simulink model "SPGF_FSK_0000_R2019b"  (R2019b)
settings: Solver=ode3  SolverName=ode4  StartTime=0.0  StopTime=1.4  FixedStep=50e-6/50  RelTol=1e-3  EnableMultiTasking=on
undefined symbols (not defined in the file): D11, Delta
libraries: powerlib x2544, powerlib_meascontrol x204, simulink x24
(part 10 of 33)

== system SPGF_FSK_0000_R2019b/TP42/Nonlinear Load ==
  Cap : powerlib/Elements/Series RLC Branch  LConnTagsString=__new0  RConnTagsString=__new0  BranchType=C  Resistance=34  Inductance=1.04  SetiL0=off  InitialCurrent=0  Capacitance=4e-06  Setx0=off  InitialVoltage=0  Measurements=None
  Cap1 : powerlib/Elements/Series RLC Branch  LConnTagsString=__new0  RConnTagsString=__new0  BranchType=C  Resistance=34  Inductance=1.04  SetiL0=off  InitialCurrent=0  Capacitance=4e-06  Setx0=off  InitialVoltage=0  Measurements=None
  Cap2 : powerlib/Elements/Series RLC Branch  LConnTagsString=__new0  RConnTagsString=__new0  BranchType=C  Resistance=34  Inductance=1.04  SetiL0=off  InitialCurrent=0  Capacitance=4e-06  Setx0=off  InitialVoltage=0  Measurements=None
  Ground : powerlib/Elements/Ground  LConnTagsString=a
  RL : powerlib/Elements/Series RLC Branch  LConnTagsString=__new0  RConnTagsString=__new0  BranchType=RL  Resistance=58  Inductance=1.04  SetiL0=off  InitialCurrent=0  Capacitance=1e-6  Setx0=off  InitialVoltage=0  Measurements=None
  RL1 : powerlib/Elements/Series RLC Branch  LConnTagsString=__new0  RConnTagsString=__new0  BranchType=RL  Resistance=40  Inductance=1.04  SetiL0=off  InitialCurrent=0  Capacitance=1e-6  Setx0=off  InitialVoltage=0  Measurements=None
  RL2 : powerlib/Elements/Series RLC Branch  LConnTagsString=__new0  RConnTagsString=__new0  BranchType=RL  Resistance=40  Inductance=1.04  SetiL0=off  InitialCurrent=0  Capacitance=1e-6  Setx0=off  InitialVoltage=0  Measurements=None
  Universal Bridge : powerlib/Power Electronics/Universal Bridge  Arms=2  SnubberResistance=1e5  SnubberCapacitance=inf  Device=Diodes  Ron=1e-3  Lon=0  ForwardVoltages="[  0  0  ]"  ForwardVoltage=-160  GTOparameters=[ 10e-6 , 20e-6 ]  IGBTparameters=[ 1e-6 , 2e-6 ]  Measurements=None  Measurements_2=None  converterType=Rectifier
  Universal Bridge1 : powerlib/Power Electronics/Universal Bridge  Arms=2  SnubberResistance=1e5  SnubberCapacitance=inf  Device=Diodes  Ron=1e-3  Lon=0  ForwardVoltages="[  0  0  ]"  ForwardVoltage=-160  GTOparameters=[ 10e-6 , 20e-6 ]  IGBTparameters=[ 1e-6 , 2e-6 ]  Measurements=None  Measurements_2=None  converterType=Rectifier
  Universal Bridge2 : powerlib/Power Electronics/Universal Bridge  Arms=2  SnubberResistance=1e5  SnubberCapacitance=inf  Device=Diodes  Ron=1e-3  Lon=0  ForwardVoltages="[  0  0  ]"  ForwardVoltage=-160  GTOparameters=[ 10e-6 , 20e-6 ]  IGBTparameters=[ 1e-6 , 2e-6 ]  Measurements=None  Measurements_2=None  converterType=Rectifier
  A : PMIOPort  Side=Left
  B : PMIOPort  Port=2  Side=Left
  C : PMIOPort  Port=3  Side=Left
  connections:
  Cap/LConn1 -- Universal Bridge/RConn1 -- RL/LConn1
  Cap/RConn1 -- RL/RConn1 -- Universal Bridge/RConn2
  Cap1/LConn1 -- Universal Bridge1/RConn1 -- RL1/LConn1
  Universal Bridge1/RConn2 -- RL1/RConn1 -- Cap1/RConn1
  Cap2/LConn1 -- Universal Bridge2/RConn1 -- RL2/LConn1
  Cap2/RConn1 -- Universal Bridge2/RConn2 -- RL2/RConn1
  Universal Bridge/LConn1 -- A/RConn1
  Universal Bridge1/LConn1 -- B/RConn1
  Universal Bridge2/LConn1 -- C/RConn1
  Ground/LConn1 -- Universal Bridge/LConn2 -- Universal Bridge1/LConn2 -- Universal Bridge2/LConn2

== system SPGF_FSK_0000_R2019b/TP42/Nonlinear Load 3ph ==
  Cap : powerlib/Elements/Series RLC Branch  LConnTagsString=__new0  RConnTagsString=__new0  BranchType=C  Resistance=34  Inductance=1.04  SetiL0=off  InitialCurrent=0  Capacitance=4e-06  Setx0=off  InitialVoltage=0  Measurements=None
  RL : powerlib/Elements/Series RLC Branch  LConnTagsString=__new0  RConnTagsString=__new0  BranchType=RL  Resistance=58  Inductance=1.04  SetiL0=off  InitialCurrent=0  Capacitance=1e-6  Setx0=off  InitialVoltage=0  Measurements=None
  Universal Bridge : powerlib/Power Electronics/Universal Bridge  Arms=3  SnubberResistance=1e5  SnubberCapacitance=inf  Device=Diodes  Ron=1e-3  Lon=0  ForwardVoltages="[  0  0  ]"  ForwardVoltage=-160  GTOparameters=[ 10e-6 , 20e-6 ]  IGBTparameters=[ 1e-6 , 2e-6 ]  Measurements=None  Measurements_2=None  converterType=Rectifier
  A : PMIOPort  Side=Left
  B : PMIOPort  Port=2  Side=Left
  C : PMIOPort  Port=3  Side=Left
  connections:
  Universal Bridge/RConn1 -- RL/LConn1 -- Cap/LConn1
  Cap/RConn1 -- Universal Bridge/RConn2 -- RL/RConn1
  Universal Bridge/LConn2 -- B/RConn1
  C/RConn1 -- Universal Bridge/LConn3
  A/RConn1 -- Universal Bridge/LConn1

== system SPGF_FSK_0000_R2019b/TP42/Q ==
  breaker : Subsystem  Commented=on  mask{SwitchA=off, SwitchB=off, SwitchC=off, InitialStatus=[1 1 1], BreakerResistance=0.0001, SnubberResistance=1e6, SnubberCapacitance=inf, TransitionTimes=[0.5 0.7], ShiftTimes=[0 0 0]}
      mask prompts: SwitchA "Switching of phase A"; SwitchB "Switching of phase B"; SwitchC "Switching of phase C"; InitialStatus "Initial status of phase breaker [A, B, C]"; BreakerResistance "Breaker resistance Ron (ohms) :"; SnubberResistance "Snubbers resistance Rp (ohms) :"; SnubberCapacitance "Snubbers capacitance Cp (F) :"; TransitionTimes "Transition times (s) :"; ShiftTimes "Time differences for switch [tA, tB, tC] (s) :"
      mask init: same as SPGF_FSK_0000_R2019b/Feed/Q/breaker
      mask Display:
      | % port_label('input',1,'Iabc');
      | 
      | port_label('lconn',1,'A');
      | port_label('lconn',2,'B');
      | port_label('lconn',3,'C');
      | 
      | port_label('rconn',1,'a');
      | port_label('rconn',2,'b');
      | port_label('rconn',3,'c');
      | 
      | disp('   Q    ');
  meas : Subsystem
  shunt : Subsystem
  A : PMIOPort  Side=Right
  B : PMIOPort  Port=2  Side=Right
  C : PMIOPort  Port=3  Side=Right
  a : PMIOPort  Port=4  Side=Left
  b : PMIOPort  Port=5  Side=Left
  c : PMIOPort  Port=6  Side=Left
  connections:
  shunt/LConn3 -- C/RConn1 -- breaker/LConn3
  shunt/LConn2 -- B/RConn1 -- breaker/LConn2
  A/RConn1 -- shunt/LConn1 -- breaker/LConn1
  meas/RConn1 -- a/RConn1
  meas/RConn2 -- b/RConn1
  meas/RConn3 -- c/RConn1
  meas/LConn3 -- breaker/RConn3 -- shunt/RConn3
  meas/LConn2 -- breaker/RConn2 -- shunt/RConn2
  meas/LConn1 -- breaker/RConn1 -- shunt/RConn1

== system SPGF_FSK_0000_R2019b/TP43/Nonlinear Load ==
  Cap : powerlib/Elements/Series RLC Branch  LConnTagsString=__new0  RConnTagsString=__new0  BranchType=C  Resistance=34  Inductance=1.04  SetiL0=off  InitialCurrent=0  Capacitance=4e-06  Setx0=off  InitialVoltage=0  Measurements=None
  Cap1 : powerlib/Elements/Series RLC Branch  LConnTagsString=__new0  RConnTagsString=__new0  BranchType=C  Resistance=34  Inductance=1.04  SetiL0=off  InitialCurrent=0  Capacitance=4e-06  Setx0=off  InitialVoltage=0  Measurements=None
  Cap2 : powerlib/Elements/Series RLC Branch  LConnTagsString=__new0  RConnTagsString=__new0  BranchType=C  Resistance=34  Inductance=1.04  SetiL0=off  InitialCurrent=0  Capacitance=4e-06  Setx0=off  InitialVoltage=0  Measurements=None
  Ground : powerlib/Elements/Ground  LConnTagsString=a
  RL : powerlib/Elements/Series RLC Branch  LConnTagsString=__new0  RConnTagsString=__new0  BranchType=RL  Resistance=58  Inductance=1.04  SetiL0=off  InitialCurrent=0  Capacitance=1e-6  Setx0=off  InitialVoltage=0  Measurements=None
  RL1 : powerlib/Elements/Series RLC Branch  LConnTagsString=__new0  RConnTagsString=__new0  BranchType=RL  Resistance=40  Inductance=1.04  SetiL0=off  InitialCurrent=0  Capacitance=1e-6  Setx0=off  InitialVoltage=0  Measurements=None
  RL2 : powerlib/Elements/Series RLC Branch  LConnTagsString=__new0  RConnTagsString=__new0  BranchType=RL  Resistance=40  Inductance=1.04  SetiL0=off  InitialCurrent=0  Capacitance=1e-6  Setx0=off  InitialVoltage=0  Measurements=None
  Universal Bridge : powerlib/Power Electronics/Universal Bridge  Arms=2  SnubberResistance=1e5  SnubberCapacitance=inf  Device=Diodes  Ron=1e-3  Lon=0  ForwardVoltages="[  0  0  ]"  ForwardVoltage=-160  GTOparameters=[ 10e-6 , 20e-6 ]  IGBTparameters=[ 1e-6 , 2e-6 ]  Measurements=None  Measurements_2=None  converterType=Rectifier
  Universal Bridge1 : powerlib/Power Electronics/Universal Bridge  Arms=2  SnubberResistance=1e5  SnubberCapacitance=inf  Device=Diodes  Ron=1e-3  Lon=0  ForwardVoltages="[  0  0  ]"  ForwardVoltage=-160  GTOparameters=[ 10e-6 , 20e-6 ]  IGBTparameters=[ 1e-6 , 2e-6 ]  Measurements=None  Measurements_2=None  converterType=Rectifier
  Universal Bridge2 : powerlib/Power Electronics/Universal Bridge  Arms=2  SnubberResistance=1e5  SnubberCapacitance=inf  Device=Diodes  Ron=1e-3  Lon=0  ForwardVoltages="[  0  0  ]"  ForwardVoltage=-160  GTOparameters=[ 10e-6 , 20e-6 ]  IGBTparameters=[ 1e-6 , 2e-6 ]  Measurements=None  Measurements_2=None  converterType=Rectifier
  A : PMIOPort  Side=Left
  B : PMIOPort  Port=2  Side=Left
  C : PMIOPort  Port=3  Side=Left
  connections:
  Cap/LConn1 -- Universal Bridge/RConn1 -- RL/LConn1
  Cap/RConn1 -- RL/RConn1 -- Universal Bridge/RConn2
  Cap1/LConn1 -- Universal Bridge1/RConn1 -- RL1/LConn1
  Universal Bridge1/RConn2 -- RL1/RConn1 -- Cap1/RConn1
  Cap2/LConn1 -- Universal Bridge2/RConn1 -- RL2/LConn1
  Cap2/RConn1 -- Universal Bridge2/RConn2 -- RL2/RConn1
  Universal Bridge/LConn1 -- A/RConn1
  Universal Bridge1/LConn1 -- B/RConn1
  Universal Bridge2/LConn1 -- C/RConn1
  Ground/LConn1 -- Universal Bridge/LConn2 -- Universal Bridge1/LConn2 -- Universal Bridge2/LConn2

== system SPGF_FSK_0000_R2019b/TP43/Nonlinear Load 3ph ==
  Cap : powerlib/Elements/Series RLC Branch  LConnTagsString=__new0  RConnTagsString=__new0  BranchType=C  Resistance=34  Inductance=1.04  SetiL0=off  InitialCurrent=0  Capacitance=4e-06  Setx0=off  InitialVoltage=0  Measurements=None
  RL : powerlib/Elements/Series RLC Branch  LConnTagsString=__new0  RConnTagsString=__new0  BranchType=RL  Resistance=58  Inductance=1.04  SetiL0=off  InitialCurrent=0  Capacitance=1e-6  Setx0=off  InitialVoltage=0  Measurements=None
  Universal Bridge : powerlib/Power Electronics/Universal Bridge  Arms=3  SnubberResistance=1e5  SnubberCapacitance=inf  Device=Diodes  Ron=1e-3  Lon=0  ForwardVoltages="[  0  0  ]"  ForwardVoltage=-160  GTOparameters=[ 10e-6 , 20e-6 ]  IGBTparameters=[ 1e-6 , 2e-6 ]  Measurements=None  Measurements_2=None  converterType=Rectifier
  A : PMIOPort  Side=Left
  B : PMIOPort  Port=2  Side=Left
  C : PMIOPort  Port=3  Side=Left
  connections:
  Universal Bridge/RConn1 -- RL/LConn1 -- Cap/LConn1
  Cap/RConn1 -- Universal Bridge/RConn2 -- RL/RConn1
  Universal Bridge/LConn2 -- B/RConn1
  C/RConn1 -- Universal Bridge/LConn3
  A/RConn1 -- Universal Bridge/LConn1

== system SPGF_FSK_0000_R2019b/TP43/Q ==
  breaker : Subsystem  Commented=on  mask{SwitchA=off, SwitchB=off, SwitchC=off, InitialStatus=[1 1 1], BreakerResistance=0.0001, SnubberResistance=1e6, SnubberCapacitance=inf, TransitionTimes=[0.5 0.7], ShiftTimes=[0 0 0]}
      mask prompts: SwitchA "Switching of phase A"; SwitchB "Switching of phase B"; SwitchC "Switching of phase C"; InitialStatus "Initial status of phase breaker [A, B, C]"; BreakerResistance "Breaker resistance Ron (ohms) :"; SnubberResistance "Snubbers resistance Rp (ohms) :"; SnubberCapacitance "Snubbers capacitance Cp (F) :"; TransitionTimes "Transition times (s) :"; ShiftTimes "Time differences for switch [tA, tB, tC] (s) :"
      mask init: same as SPGF_FSK_0000_R2019b/Feed/Q/breaker
      mask Display:
      | % port_label('input',1,'Iabc');
      | 
      | port_label('lconn',1,'A');
      | port_label('lconn',2,'B');
      | port_label('lconn',3,'C');
      | 
      | port_label('rconn',1,'a');
      | port_label('rconn',2,'b');
      | port_label('rconn',3,'c');
      | 
      | disp('   Q    ');
  meas : Subsystem
  shunt : Subsystem
  A : PMIOPort  Side=Right
  B : PMIOPort  Port=2  Side=Right
  C : PMIOPort  Port=3  Side=Right
  a : PMIOPort  Port=4  Side=Left
  b : PMIOPort  Port=5  Side=Left
  c : PMIOPort  Port=6  Side=Left
  connections:
  shunt/LConn3 -- C/RConn1 -- breaker/LConn3
  shunt/LConn2 -- B/RConn1 -- breaker/LConn2
  A/RConn1 -- shunt/LConn1 -- breaker/LConn1
  meas/RConn1 -- a/RConn1
  meas/RConn2 -- b/RConn1
  meas/RConn3 -- c/RConn1
  meas/LConn3 -- breaker/RConn3 -- shunt/RConn3
  meas/LConn2 -- breaker/RConn2 -- shunt/RConn2
  meas/LConn1 -- breaker/RConn1 -- shunt/RConn1

== system SPGF_FSK_0000_R2019b/TP51/Nonlinear Load ==
  Cap : powerlib/Elements/Series RLC Branch  LConnTagsString=__new0  RConnTagsString=__new0  BranchType=C  Resistance=34  Inductance=1.04  SetiL0=off  InitialCurrent=0  Capacitance=4e-06  Setx0=off  InitialVoltage=0  Measurements=None
  Cap1 : powerlib/Elements/Series RLC Branch  LConnTagsString=__new0  RConnTagsString=__new0  BranchType=C  Resistance=34  Inductance=1.04  SetiL0=off  InitialCurrent=0  Capacitance=4e-06  Setx0=off  InitialVoltage=0  Measurements=None
  Cap2 : powerlib/Elements/Series RLC Branch  LConnTagsString=__new0  RConnTagsString=__new0  BranchType=C  Resistance=34  Inductance=1.04  SetiL0=off  InitialCurrent=0  Capacitance=4e-06  Setx0=off  InitialVoltage=0  Measurements=None
  Ground : powerlib/Elements/Ground  LConnTagsString=a
  RL : powerlib/Elements/Series RLC Branch  LConnTagsString=__new0  RConnTagsString=__new0  BranchType=RL  Resistance=58  Inductance=1.04  SetiL0=off  InitialCurrent=0  Capacitance=1e-6  Setx0=off  InitialVoltage=0  Measurements=None
  RL1 : powerlib/Elements/Series RLC Branch  LConnTagsString=__new0  RConnTagsString=__new0  BranchType=RL  Resistance=40  Inductance=1.04  SetiL0=off  InitialCurrent=0  Capacitance=1e-6  Setx0=off  InitialVoltage=0  Measurements=None
  RL2 : powerlib/Elements/Series RLC Branch  LConnTagsString=__new0  RConnTagsString=__new0  BranchType=RL  Resistance=40  Inductance=1.04  SetiL0=off  InitialCurrent=0  Capacitance=1e-6  Setx0=off  InitialVoltage=0  Measurements=None
  Universal Bridge : powerlib/Power Electronics/Universal Bridge  Arms=2  SnubberResistance=1e5  SnubberCapacitance=inf  Device=Diodes  Ron=1e-3  Lon=0  ForwardVoltages="[  0  0  ]"  ForwardVoltage=-160  GTOparameters=[ 10e-6 , 20e-6 ]  IGBTparameters=[ 1e-6 , 2e-6 ]  Measurements=None  Measurements_2=None  converterType=Rectifier
  Universal Bridge1 : powerlib/Power Electronics/Universal Bridge  Arms=2  SnubberResistance=1e5  SnubberCapacitance=inf  Device=Diodes  Ron=1e-3  Lon=0  ForwardVoltages="[  0  0  ]"  ForwardVoltage=-160  GTOparameters=[ 10e-6 , 20e-6 ]  IGBTparameters=[ 1e-6 , 2e-6 ]  Measurements=None  Measurements_2=None  converterType=Rectifier
  Universal Bridge2 : powerlib/Power Electronics/Universal Bridge  Arms=2  SnubberResistance=1e5  SnubberCapacitance=inf  Device=Diodes  Ron=1e-3  Lon=0  ForwardVoltages="[  0  0  ]"  ForwardVoltage=-160  GTOparameters=[ 10e-6 , 20e-6 ]  IGBTparameters=[ 1e-6 , 2e-6 ]  Measurements=None  Measurements_2=None  converterType=Rectifier
  A : PMIOPort  Side=Left
  B : PMIOPort  Port=2  Side=Left
  C : PMIOPort  Port=3  Side=Left
  connections:
  Cap/LConn1 -- Universal Bridge/RConn1 -- RL/LConn1
  Cap/RConn1 -- RL/RConn1 -- Universal Bridge/RConn2
  Cap1/LConn1 -- Universal Bridge1/RConn1 -- RL1/LConn1
  Universal Bridge1/RConn2 -- RL1/RConn1 -- Cap1/RConn1
  Cap2/LConn1 -- Universal Bridge2/RConn1 -- RL2/LConn1
  Cap2/RConn1 -- Universal Bridge2/RConn2 -- RL2/RConn1
  Universal Bridge/LConn1 -- A/RConn1
  Universal Bridge1/LConn1 -- B/RConn1
  Universal Bridge2/LConn1 -- C/RConn1
  Ground/LConn1 -- Universal Bridge/LConn2 -- Universal Bridge1/LConn2 -- Universal Bridge2/LConn2

== system SPGF_FSK_0000_R2019b/TP51/Nonlinear Load 3ph ==
  Cap : powerlib/Elements/Series RLC Branch  LConnTagsString=__new0  RConnTagsString=__new0  BranchType=C  Resistance=34  Inductance=1.04  SetiL0=off  InitialCurrent=0  Capacitance=4e-06  Setx0=off  InitialVoltage=0  Measurements=None
  RL : powerlib/Elements/Series RLC Branch  LConnTagsString=__new0  RConnTagsString=__new0  BranchType=RL  Resistance=58  Inductance=1.04  SetiL0=off  InitialCurrent=0  Capacitance=1e-6  Setx0=off  InitialVoltage=0  Measurements=None
  Universal Bridge : powerlib/Power Electronics/Universal Bridge  Arms=3  SnubberResistance=1e5  SnubberCapacitance=inf  Device=Diodes  Ron=1e-3  Lon=0  ForwardVoltages="[  0  0  ]"  ForwardVoltage=-160  GTOparameters=[ 10e-6 , 20e-6 ]  IGBTparameters=[ 1e-6 , 2e-6 ]  Measurements=None  Measurements_2=None  converterType=Rectifier
  A : PMIOPort  Side=Left
  B : PMIOPort  Port=2  Side=Left
  C : PMIOPort  Port=3  Side=Left
  connections:
  Universal Bridge/RConn1 -- RL/LConn1 -- Cap/LConn1
  Cap/RConn1 -- Universal Bridge/RConn2 -- RL/RConn1
  Universal Bridge/LConn2 -- B/RConn1
  C/RConn1 -- Universal Bridge/LConn3
  A/RConn1 -- Universal Bridge/LConn1

== system SPGF_FSK_0000_R2019b/TP51/Q ==
  breaker : Subsystem  Commented=on  mask{SwitchA=off, SwitchB=off, SwitchC=off, InitialStatus=[1 1 1], BreakerResistance=0.0001, SnubberResistance=1e6, SnubberCapacitance=inf, TransitionTimes=[0.5 0.7], ShiftTimes=[0 0 0]}
      mask prompts: SwitchA "Switching of phase A"; SwitchB "Switching of phase B"; SwitchC "Switching of phase C"; InitialStatus "Initial status of phase breaker [A, B, C]"; BreakerResistance "Breaker resistance Ron (ohms) :"; SnubberResistance "Snubbers resistance Rp (ohms) :"; SnubberCapacitance "Snubbers capacitance Cp (F) :"; TransitionTimes "Transition times (s) :"; ShiftTimes "Time differences for switch [tA, tB, tC] (s) :"
      mask init: same as SPGF_FSK_0000_R2019b/Feed/Q/breaker
      mask Display:
      | % port_label('input',1,'Iabc');
      | 
      | port_label('lconn',1,'A');
      | port_label('lconn',2,'B');
      | port_label('lconn',3,'C');
      | 
      | port_label('rconn',1,'a');
      | port_label('rconn',2,'b');
      | port_label('rconn',3,'c');
      | 
      | disp('   Q    ');
  meas : Subsystem
  shunt : Subsystem
  A : PMIOPort  Side=Right
  B : PMIOPort  Port=2  Side=Right
  C : PMIOPort  Port=3  Side=Right
  a : PMIOPort  Port=4  Side=Left
  b : PMIOPort  Port=5  Side=Left
  c : PMIOPort  Port=6  Side=Left
  connections:
  shunt/LConn3 -- C/RConn1 -- breaker/LConn3
  shunt/LConn2 -- B/RConn1 -- breaker/LConn2
  A/RConn1 -- shunt/LConn1 -- breaker/LConn1
  meas/RConn1 -- a/RConn1
  meas/RConn2 -- b/RConn1
  meas/RConn3 -- c/RConn1
  meas/LConn3 -- breaker/RConn3 -- shunt/RConn3
  meas/LConn2 -- breaker/RConn2 -- shunt/RConn2
  meas/LConn1 -- breaker/RConn1 -- shunt/RConn1

== system SPGF_FSK_0000_R2019b/TP52/Nonlinear Load ==
  Cap : powerlib/Elements/Series RLC Branch  LConnTagsString=__new0  RConnTagsString=__new0  BranchType=C  Resistance=34  Inductance=1.04  SetiL0=off  InitialCurrent=0  Capacitance=4e-06  Setx0=off  InitialVoltage=0  Measurements=None
  Cap1 : powerlib/Elements/Series RLC Branch  LConnTagsString=__new0  RConnTagsString=__new0  BranchType=C  Resistance=34  Inductance=1.04  SetiL0=off  InitialCurrent=0  Capacitance=4e-06  Setx0=off  InitialVoltage=0  Measurements=None
  Cap2 : powerlib/Elements/Series RLC Branch  LConnTagsString=__new0  RConnTagsString=__new0  BranchType=C  Resistance=34  Inductance=1.04  SetiL0=off  InitialCurrent=0  Capacitance=4e-06  Setx0=off  InitialVoltage=0  Measurements=None
  Ground : powerlib/Elements/Ground  LConnTagsString=a
  RL : powerlib/Elements/Series RLC Branch  LConnTagsString=__new0  RConnTagsString=__new0  BranchType=RL  Resistance=58  Inductance=1.04  SetiL0=off  InitialCurrent=0  Capacitance=1e-6  Setx0=off  InitialVoltage=0  Measurements=None
  RL1 : powerlib/Elements/Series RLC Branch  LConnTagsString=__new0  RConnTagsString=__new0  BranchType=RL  Resistance=40  Inductance=1.04  SetiL0=off  InitialCurrent=0  Capacitance=1e-6  Setx0=off  InitialVoltage=0  Measurements=None
  RL2 : powerlib/Elements/Series RLC Branch  LConnTagsString=__new0  RConnTagsString=__new0  BranchType=RL  Resistance=40  Inductance=1.04  SetiL0=off  InitialCurrent=0  Capacitance=1e-6  Setx0=off  InitialVoltage=0  Measurements=None
  Universal Bridge : powerlib/Power Electronics/Universal Bridge  Arms=2  SnubberResistance=1e5  SnubberCapacitance=inf  Device=Diodes  Ron=1e-3  Lon=0  ForwardVoltages="[  0  0  ]"  ForwardVoltage=-160  GTOparameters=[ 10e-6 , 20e-6 ]  IGBTparameters=[ 1e-6 , 2e-6 ]  Measurements=None  Measurements_2=None  converterType=Rectifier
  Universal Bridge1 : powerlib/Power Electronics/Universal Bridge  Arms=2  SnubberResistance=1e5  SnubberCapacitance=inf  Device=Diodes  Ron=1e-3  Lon=0  ForwardVoltages="[  0  0  ]"  ForwardVoltage=-160  GTOparameters=[ 10e-6 , 20e-6 ]  IGBTparameters=[ 1e-6 , 2e-6 ]  Measurements=None  Measurements_2=None  converterType=Rectifier
  Universal Bridge2 : powerlib/Power Electronics/Universal Bridge  Arms=2  SnubberResistance=1e5  SnubberCapacitance=inf  Device=Diodes  Ron=1e-3  Lon=0  ForwardVoltages="[  0  0  ]"  ForwardVoltage=-160  GTOparameters=[ 10e-6 , 20e-6 ]  IGBTparameters=[ 1e-6 , 2e-6 ]  Measurements=None  Measurements_2=None  converterType=Rectifier
  A : PMIOPort  Side=Left
  B : PMIOPort  Port=2  Side=Left
  C : PMIOPort  Port=3  Side=Left
  connections:
  Cap/LConn1 -- Universal Bridge/RConn1 -- RL/LConn1
  Cap/RConn1 -- RL/RConn1 -- Universal Bridge/RConn2
  Cap1/LConn1 -- Universal Bridge1/RConn1 -- RL1/LConn1
  Universal Bridge1/RConn2 -- RL1/RConn1 -- Cap1/RConn1
  Cap2/LConn1 -- Universal Bridge2/RConn1 -- RL2/LConn1
  Cap2/RConn1 -- Universal Bridge2/RConn2 -- RL2/RConn1
  Universal Bridge/LConn1 -- A/RConn1
  Universal Bridge1/LConn1 -- B/RConn1
  Universal Bridge2/LConn1 -- C/RConn1
  Ground/LConn1 -- Universal Bridge/LConn2 -- Universal Bridge1/LConn2 -- Universal Bridge2/LConn2

== system SPGF_FSK_0000_R2019b/TP52/Nonlinear Load 3ph ==
  Cap : powerlib/Elements/Series RLC Branch  LConnTagsString=__new0  RConnTagsString=__new0  BranchType=C  Resistance=34  Inductance=1.04  SetiL0=off  InitialCurrent=0  Capacitance=4e-06  Setx0=off  InitialVoltage=0  Measurements=None
  RL : powerlib/Elements/Series RLC Branch  LConnTagsString=__new0  RConnTagsString=__new0  BranchType=RL  Resistance=58  Inductance=1.04  SetiL0=off  InitialCurrent=0  Capacitance=1e-6  Setx0=off  InitialVoltage=0  Measurements=None
  Universal Bridge : powerlib/Power Electronics/Universal Bridge  Arms=3  SnubberResistance=1e5  SnubberCapacitance=inf  Device=Diodes  Ron=1e-3  Lon=0  ForwardVoltages="[  0  0  ]"  ForwardVoltage=-160  GTOparameters=[ 10e-6 , 20e-6 ]  IGBTparameters=[ 1e-6 , 2e-6 ]  Measurements=None  Measurements_2=None  converterType=Rectifier
  A : PMIOPort  Side=Left
  B : PMIOPort  Port=2  Side=Left
  C : PMIOPort  Port=3  Side=Left
  connections:
  Universal Bridge/RConn1 -- RL/LConn1 -- Cap/LConn1
  Cap/RConn1 -- Universal Bridge/RConn2 -- RL/RConn1
  Universal Bridge/LConn2 -- B/RConn1
  C/RConn1 -- Universal Bridge/LConn3
  A/RConn1 -- Universal Bridge/LConn1

== system SPGF_FSK_0000_R2019b/TP52/Q ==
  breaker : Subsystem  Commented=on  mask{SwitchA=off, SwitchB=off, SwitchC=off, InitialStatus=[1 1 1], BreakerResistance=0.0001, SnubberResistance=1e6, SnubberCapacitance=inf, TransitionTimes=[0.5 0.7], ShiftTimes=[0 0 0]}
      mask prompts: SwitchA "Switching of phase A"; SwitchB "Switching of phase B"; SwitchC "Switching of phase C"; InitialStatus "Initial status of phase breaker [A, B, C]"; BreakerResistance "Breaker resistance Ron (ohms) :"; SnubberResistance "Snubbers resistance Rp (ohms) :"; SnubberCapacitance "Snubbers capacitance Cp (F) :"; TransitionTimes "Transition times (s) :"; ShiftTimes "Time differences for switch [tA, tB, tC] (s) :"
      mask init: same as SPGF_FSK_0000_R2019b/Feed/Q/breaker
      mask Display:
      | % port_label('input',1,'Iabc');
      | 
      | port_label('lconn',1,'A');
      | port_label('lconn',2,'B');
      | port_label('lconn',3,'C');
      | 
      | port_label('rconn',1,'a');
      | port_label('rconn',2,'b');
      | port_label('rconn',3,'c');
      | 
      | disp('   Q    ');
  meas : Subsystem
  shunt : Subsystem
  A : PMIOPort  Side=Right
  B : PMIOPort  Port=2  Side=Right
  C : PMIOPort  Port=3  Side=Right
  a : PMIOPort  Port=4  Side=Left
  b : PMIOPort  Port=5  Side=Left
  c : PMIOPort  Port=6  Side=Left
  connections:
  shunt/LConn3 -- C/RConn1 -- breaker/LConn3
  shunt/LConn2 -- B/RConn1 -- breaker/LConn2
  A/RConn1 -- shunt/LConn1 -- breaker/LConn1
  meas/RConn1 -- a/RConn1
  meas/RConn2 -- b/RConn1
  meas/RConn3 -- c/RConn1
  meas/LConn3 -- breaker/RConn3 -- shunt/RConn3
  meas/LConn2 -- breaker/RConn2 -- shunt/RConn2
  meas/LConn1 -- breaker/RConn1 -- shunt/RConn1

== system SPGF_FSK_0000_R2019b/TP53/Nonlinear Load ==
  Cap : powerlib/Elements/Series RLC Branch  LConnTagsString=__new0  RConnTagsString=__new0  BranchType=C  Resistance=34  Inductance=1.04  SetiL0=off  InitialCurrent=0  Capacitance=4e-06  Setx0=off  InitialVoltage=0  Measurements=None
  Cap1 : powerlib/Elements/Series RLC Branch  LConnTagsString=__new0  RConnTagsString=__new0  BranchType=C  Resistance=34  Inductance=1.04  SetiL0=off  InitialCurrent=0  Capacitance=4e-06  Setx0=off  InitialVoltage=0  Measurements=None
  Cap2 : powerlib/Elements/Series RLC Branch  LConnTagsString=__new0  RConnTagsString=__new0  BranchType=C  Resistance=34  Inductance=1.04  SetiL0=off  InitialCurrent=0  Capacitance=4e-06  Setx0=off  InitialVoltage=0  Measurements=None
  Ground : powerlib/Elements/Ground  LConnTagsString=a
  RL : powerlib/Elements/Series RLC Branch  LConnTagsString=__new0  RConnTagsString=__new0  BranchType=RL  Resistance=58  Inductance=1.04  SetiL0=off  InitialCurrent=0  Capacitance=1e-6  Setx0=off  InitialVoltage=0  Measurements=None
  RL1 : powerlib/Elements/Series RLC Branch  LConnTagsString=__new0  RConnTagsString=__new0  BranchType=RL  Resistance=40  Inductance=1.04  SetiL0=off  InitialCurrent=0  Capacitance=1e-6  Setx0=off  InitialVoltage=0  Measurements=None
  RL2 : powerlib/Elements/Series RLC Branch  LConnTagsString=__new0  RConnTagsString=__new0  BranchType=RL  Resistance=40  Inductance=1.04  SetiL0=off  InitialCurrent=0  Capacitance=1e-6  Setx0=off  InitialVoltage=0  Measurements=None
  Universal Bridge : powerlib/Power Electronics/Universal Bridge  Arms=2  SnubberResistance=1e5  SnubberCapacitance=inf  Device=Diodes  Ron=1e-3  Lon=0  ForwardVoltages="[  0  0  ]"  ForwardVoltage=-160  GTOparameters=[ 10e-6 , 20e-6 ]  IGBTparameters=[ 1e-6 , 2e-6 ]  Measurements=None  Measurements_2=None  converterType=Rectifier
  Universal Bridge1 : powerlib/Power Electronics/Universal Bridge  Arms=2  SnubberResistance=1e5  SnubberCapacitance=inf  Device=Diodes  Ron=1e-3  Lon=0  ForwardVoltages="[  0  0  ]"  ForwardVoltage=-160  GTOparameters=[ 10e-6 , 20e-6 ]  IGBTparameters=[ 1e-6 , 2e-6 ]  Measurements=None  Measurements_2=None  converterType=Rectifier
  Universal Bridge2 : powerlib/Power Electronics/Universal Bridge  Arms=2  SnubberResistance=1e5  SnubberCapacitance=inf  Device=Diodes  Ron=1e-3  Lon=0  ForwardVoltages="[  0  0  ]"  ForwardVoltage=-160  GTOparameters=[ 10e-6 , 20e-6 ]  IGBTparameters=[ 1e-6 , 2e-6 ]  Measurements=None  Measurements_2=None  converterType=Rectifier
  A : PMIOPort  Side=Left
  B : PMIOPort  Port=2  Side=Left
  C : PMIOPort  Port=3  Side=Left
  connections:
  Cap/LConn1 -- Universal Bridge/RConn1 -- RL/LConn1
  Cap/RConn1 -- RL/RConn1 -- Universal Bridge/RConn2
  Cap1/LConn1 -- Universal Bridge1/RConn1 -- RL1/LConn1
  Universal Bridge1/RConn2 -- RL1/RConn1 -- Cap1/RConn1
  Cap2/LConn1 -- Universal Bridge2/RConn1 -- RL2/LConn1
  Cap2/RConn1 -- Universal Bridge2/RConn2 -- RL2/RConn1
  Universal Bridge/LConn1 -- A/RConn1
  Universal Bridge1/LConn1 -- B/RConn1
  Universal Bridge2/LConn1 -- C/RConn1
  Ground/LConn1 -- Universal Bridge/LConn2 -- Universal Bridge1/LConn2 -- Universal Bridge2/LConn2

== system SPGF_FSK_0000_R2019b/TP53/Nonlinear Load 3ph ==
  Cap : powerlib/Elements/Series RLC Branch  LConnTagsString=__new0  RConnTagsString=__new0  BranchType=C  Resistance=34  Inductance=1.04  SetiL0=off  InitialCurrent=0  Capacitance=4e-06  Setx0=off  InitialVoltage=0  Measurements=None
  RL : powerlib/Elements/Series RLC Branch  LConnTagsString=__new0  RConnTagsString=__new0  BranchType=RL  Resistance=58  Inductance=1.04  SetiL0=off  InitialCurrent=0  Capacitance=1e-6  Setx0=off  InitialVoltage=0  Measurements=None
  Universal Bridge : powerlib/Power Electronics/Universal Bridge  Arms=3  SnubberResistance=1e5  SnubberCapacitance=inf  Device=Diodes  Ron=1e-3  Lon=0  ForwardVoltages="[  0  0  ]"  ForwardVoltage=-160  GTOparameters=[ 10e-6 , 20e-6 ]  IGBTparameters=[ 1e-6 , 2e-6 ]  Measurements=None  Measurements_2=None  converterType=Rectifier
  A : PMIOPort  Side=Left
  B : PMIOPort  Port=2  Side=Left
  C : PMIOPort  Port=3  Side=Left
  connections:
  Universal Bridge/RConn1 -- RL/LConn1 -- Cap/LConn1
  Cap/RConn1 -- Universal Bridge/RConn2 -- RL/RConn1
  Universal Bridge/LConn2 -- B/RConn1
  C/RConn1 -- Universal Bridge/LConn3
  A/RConn1 -- Universal Bridge/LConn1

== system SPGF_FSK_0000_R2019b/TP53/Q ==
  breaker : Subsystem  Commented=on  mask{SwitchA=off, SwitchB=off, SwitchC=off, InitialStatus=[1 1 1], BreakerResistance=0.0001, SnubberResistance=1e6, SnubberCapacitance=inf, TransitionTimes=[0.5 0.7], ShiftTimes=[0 0 0]}
      mask prompts: SwitchA "Switching of phase A"; SwitchB "Switching of phase B"; SwitchC "Switching of phase C"; InitialStatus "Initial status of phase breaker [A, B, C]"; BreakerResistance "Breaker resistance Ron (ohms) :"; SnubberResistance "Snubbers resistance Rp (ohms) :"; SnubberCapacitance "Snubbers capacitance Cp (F) :"; TransitionTimes "Transition times (s) :"; ShiftTimes "Time differences for switch [tA, tB, tC] (s) :"
      mask init: same as SPGF_FSK_0000_R2019b/Feed/Q/breaker
      mask Display:
      | % port_label('input',1,'Iabc');
      | 
      | port_label('lconn',1,'A');
      | port_label('lconn',2,'B');
      | port_label('lconn',3,'C');
      | 
      | port_label('rconn',1,'a');
      | port_label('rconn',2,'b');
      | port_label('rconn',3,'c');
      | 
      | disp('   Q    ');
  meas : Subsystem
  shunt : Subsystem
  A : PMIOPort  Side=Right
  B : PMIOPort  Port=2  Side=Right
  C : PMIOPort  Port=3  Side=Right
  a : PMIOPort  Port=4  Side=Left
  b : PMIOPort  Port=5  Side=Left
  c : PMIOPort  Port=6  Side=Left
  connections:
  shunt/LConn3 -- C/RConn1 -- breaker/LConn3
  shunt/LConn2 -- B/RConn1 -- breaker/LConn2
  A/RConn1 -- shunt/LConn1 -- breaker/LConn1
  meas/RConn1 -- a/RConn1
  meas/RConn2 -- b/RConn1
  meas/RConn3 -- c/RConn1
  meas/LConn3 -- breaker/RConn3 -- shunt/RConn3
  meas/LConn2 -- breaker/RConn2 -- shunt/RConn2
  meas/LConn1 -- breaker/RConn1 -- shunt/RConn1

== system SPGF_FSK_0000_R2019b/TSN/DGR ==
  Current Measurement : powerlib/Measurements/Current Measurement  PhasorSimulation=off  OutputType=Complex  PSBequivalent=0
  Fourier : powerlib_meascontrol/Measurements/Fourier  Freq=50  n=1  InInit=[0, 0]  Ts=0
  Fourier1 : powerlib_meascontrol/Measurements/Fourier  Freq=50  n=1  InInit=[0, 0]  Ts=0
  Gain : Gain  Gain=1/sqrt(2)
  Ground1 : powerlib/Elements/Ground  LConnTagsString=a
  RmL : powerlib/Elements/Series RLC Branch  LConnTagsString=__new0  RConnTagsString=__new0  BranchType=RL  Resistance=Rm  Inductance=L  SetiL0=off  InitialCurrent=0  Capacitance=1e-6  Setx0=off  InitialVoltage=0  Measurements=None
  Rst : powerlib/Elements/Series RLC Branch  LConnTagsString=__new0  RConnTagsString=__new0  BranchType=R  Resistance=Rst  Inductance=1000e-3  SetiL0=off  InitialCurrent=0  Capacitance=1e-6  Setx0=off  InitialVoltage=0  Measurements=None
  Scope : Scope  NumInputPorts=2
  Scope1 : Scope  NumInputPorts=2
  Voltage Measurement : powerlib/Measurements/Voltage Measurement  PhasorSimulation=off  OutputType=Complex  PSBequivalent=0
  N : PMIOPort  Side=Right
  wires:
  Gain/1 -> Scope/1
  Fourier/1 -> Gain/1
  Voltage Measurement/1 -> Fourier/1, Scope1/1
  Current Measurement/1 -> Fourier1/1, Scope1/2
  Fourier1/1 -> Scope/2
  connections:
  RmL/LConn1 -- Current Measurement/LConn1 -- Voltage Measurement/LConn2 -- Rst/LConn1
  RmL/RConn1 -- Rst/RConn1 -- Voltage Measurement/LConn1 -- N/RConn1
  Current Measurement/RConn1 -- Ground1/LConn1

== system SPGF_FSK_0000_R2019b/V1/VT ==
  Ground3 : powerlib/Elements/Ground  LConnTagsString=a
  Ground4 : powerlib/Elements/Ground  LConnTagsString=a
  Ground5 : powerlib/Elements/Ground  LConnTagsString=a
  Mux2 : Mux  Inputs=3
  Mux3 : Mux  Inputs=3
  R Load A1 : powerlib/Elements/Series RLC Load  LConnTagsString=a  RConnTagsString=__new0  NominalVoltage=57.735  NominalFrequency=50  ActivePower=150  InductivePower=0  CapacitivePower=0  Setx0=off  InitialVoltage=0  SetiL0=off  InitialCurrent=0  Measurements=None  LoadType=constant Z
  R Load B1 : powerlib/Elements/Series RLC Load  LConnTagsString=a  RConnTagsString=__new0  NominalVoltage=57.735  NominalFrequency=50  ActivePower=150  InductivePower=0  CapacitivePower=0  Setx0=off  InitialVoltage=0  SetiL0=off  InitialCurrent=0  Measurements=None  LoadType=constant Z
  R Load C1 : powerlib/Elements/Series RLC Load  LConnTagsString=a  RConnTagsString=__new0  NominalVoltage=57.735  NominalFrequency=50  ActivePower=150  InductivePower=0  CapacitivePower=0  Setx0=off  InitialVoltage=0  SetiL0=off  InitialCurrent=0  Measurements=None  LoadType=constant Z
  U A:3 : powerlib/Measurements/Voltage Measurement  PhasorSimulation=off  OutputType=Complex  PSBequivalent=0
  U A:4 : powerlib/Measurements/Voltage Measurement  PhasorSimulation=off  OutputType=Complex  PSBequivalent=0
  U B:3 : powerlib/Measurements/Voltage Measurement  PhasorSimulation=off  OutputType=Complex  PSBequivalent=0
  U B:4 : powerlib/Measurements/Voltage Measurement  PhasorSimulation=off  OutputType=Complex  PSBequivalent=0
  U C:3 : powerlib/Measurements/Voltage Measurement  PhasorSimulation=off  OutputType=Complex  PSBequivalent=0
  U C:4 : powerlib/Measurements/Voltage Measurement  PhasorSimulation=off  OutputType=Complex  PSBequivalent=0
  U0:1 : powerlib/Measurements/Voltage Measurement  PhasorSimulation=off  OutputType=Complex  PSBequivalent=0
  VT A1 : powerlib/Elements/Saturable Transformer  ThreeWindings=on  Hysteresis=off  DataFile='hysteresis.mat'  Measurements=None  UNITS=pu  NominalPower=[600, 50]  Winding1=[5773.503, 0.00562500, 0.02315000]  Winding2=[57.735, 0.00562500, 0.02315000]  Winding3=[33.333, 0.00010000, 0.00010000]  Saturation=[ 0,0 ; 0.0024,1.2 ; 1.0,1.52 ]  CoreLoss=[500]  BreakLoop=on  DiscreteSolver=Trapezoidal iterative  DataType=off  InitialFlux=-24.7391768751303  TransfoNumber=1
  VT B1 : powerlib/Elements/Saturable Transformer  ThreeWindings=on  Hysteresis=off  DataFile='hysteresis.mat'  Measurements=None  UNITS=pu  NominalPower=[600, 50]  Winding1=[5773.503, 0.00562500, 0.02315000]  Winding2=[57.735, 0.00562500, 0.02315000]  Winding3=[33.333, 0.00010000, 0.00010000]  Saturation=[ 0,0 ; 0.0024,1.2 ; 1.0,1.52 ]  CoreLoss=[500]  BreakLoop=on  DiscreteSolver=Trapezoidal iterative  DataType=off  InitialFlux=0.446625542508336  TransfoNumber=1
  VT C1 : powerlib/Elements/Saturable Transformer  ThreeWindings=on  Hysteresis=off  DataFile='hysteresis.mat'  Measurements=None  UNITS=pu  NominalPower=[600, 50]  Winding1=[5773.503, 0.00562500, 0.02315000]  Winding2=[57.735, 0.00562500, 0.02315000]  Winding3=[33.333, 0.00010000, 0.00010000]  Saturation=[ 0,0 ; 0.0024,1.2 ; 1.0,1.52 ]  CoreLoss=[500]  BreakLoop=on  DiscreteSolver=Trapezoidal iterative  DataType=off  InitialFlux=24.2925513332878  TransfoNumber=1
  A : PMIOPort  Side=Left
  B : PMIOPort  Port=2  Side=Left
  C : PMIOPort  Port=3  Side=Left
  Uabc1 : Outport
  Uabc2 : Outport  Port=2
  3U0 : Outport  Port=3
  wires:
  Mux3/1 -> Uabc2/1
  U0:1/1 -> 3U0/1
  Mux2/1 -> Uabc1/1
  U C:4/1 -> Mux3/3
  U B:4/1 -> Mux3/2
  U A:4/1 -> Mux3/1
  U C:3/1 -> Mux2/3
  U B:3/1 -> Mux2/2
  U A:3/1 -> Mux2/1
  connections:
  U0:1/LConn2 -- Ground4/LConn1 -- VT C1/RConn4
  VT B1/RConn2 -- VT A1/RConn2 -- U A:4/LConn2 -- U B:4/LConn2 -- U C:4/LConn2 -- R Load A1/RConn1 -- R Load B1/RConn1 -- R Load C1/RConn1 -- VT C1/RConn2
  R Load B1/LConn1 -- U B:4/LConn1 -- VT B1/RConn1
  R Load C1/LConn1 -- U C:4/LConn1 -- VT C1/RConn1
  U B:3/LConn1 -- B/RConn1 -- VT B1/LConn1
  U C:3/LConn1 -- C/RConn1 -- VT C1/LConn1
  R Load A1/LConn1 -- U A:4/LConn1 -- VT A1/RConn1
  VT A1/LConn1 -- A/RConn1 -- U A:3/LConn1
  U A:3/LConn2 -- VT A1/LConn2 -- VT B1/LConn2 -- U B:3/LConn2 -- VT C1/LConn2 -- Ground3/LConn1 -- U C:3/LConn2
  VT B1/RConn4 -- VT C1/RConn3
  VT A1/RConn3 -- U0:1/LConn1
  VT A1/RConn4 -- VT B1/RConn3

== system SPGF_FSK_0000_R2019b/V53/VT ==
  Ground3 : powerlib/Elements/Ground  LConnTagsString=a
  Ground4 : powerlib/Elements/Ground  LConnTagsString=a
  Ground5 : powerlib/Elements/Ground  LConnTagsString=a
  Mux2 : Mux  Inputs=3
  Mux3 : Mux  Inputs=3
  R Load A1 : powerlib/Elements/Series RLC Load  LConnTagsString=a  RConnTagsString=__new0  NominalVoltage=57.735  NominalFrequency=50  ActivePower=150  InductivePower=0  CapacitivePower=0  Setx0=off  InitialVoltage=0  SetiL0=off  InitialCurrent=0  Measurements=None  LoadType=constant Z
  R Load B1 : powerlib/Elements/Series RLC Load  LConnTagsString=a  RConnTagsString=__new0  NominalVoltage=57.735  NominalFrequency=50  ActivePower=150  InductivePower=0  CapacitivePower=0  Setx0=off  InitialVoltage=0  SetiL0=off  InitialCurrent=0  Measurements=None  LoadType=constant Z
  R Load C1 : powerlib/Elements/Series RLC Load  LConnTagsString=a  RConnTagsString=__new0  NominalVoltage=57.735  NominalFrequency=50  ActivePower=150  InductivePower=0  CapacitivePower=0  Setx0=off  InitialVoltage=0  SetiL0=off  InitialCurrent=0  Measurements=None  LoadType=constant Z
  U A:3 : powerlib/Measurements/Voltage Measurement  PhasorSimulation=off  OutputType=Complex  PSBequivalent=0
  U A:4 : powerlib/Measurements/Voltage Measurement  PhasorSimulation=off  OutputType=Complex  PSBequivalent=0
  U B:3 : powerlib/Measurements/Voltage Measurement  PhasorSimulation=off  OutputType=Complex  PSBequivalent=0
  U B:4 : powerlib/Measurements/Voltage Measurement  PhasorSimulation=off  OutputType=Complex  PSBequivalent=0
  U C:3 : powerlib/Measurements/Voltage Measurement  PhasorSimulation=off  OutputType=Complex  PSBequivalent=0
  U C:4 : powerlib/Measurements/Voltage Measurement  PhasorSimulation=off  OutputType=Complex  PSBequivalent=0
  U0:1 : powerlib/Measurements/Voltage Measurement  PhasorSimulation=off  OutputType=Complex  PSBequivalent=0
  VT A1 : powerlib/Elements/Saturable Transformer  ThreeWindings=on  Hysteresis=off  DataFile='hysteresis.mat'  Measurements=None  UNITS=pu  NominalPower=[600, 50]  Winding1=[5773.503, 0.00562500, 0.02315000]  Winding2=[57.735, 0.00562500, 0.02315000]  Winding3=[33.333, 0.00010000, 0.00010000]  Saturation=[ 0,0 ; 0.0024,1.2 ; 1.0,1.52 ]  CoreLoss=[500]  BreakLoop=on  DiscreteSolver=Trapezoidal iterative  DataType=off  InitialFlux=-24.6148264896066  TransfoNumber=1
  VT B1 : powerlib/Elements/Saturable Transformer  ThreeWindings=on  Hysteresis=off  DataFile='hysteresis.mat'  Measurements=None  UNITS=pu  NominalPower=[600, 50]  Winding1=[5773.503, 0.00562500, 0.02315000]  Winding2=[57.735, 0.00562500, 0.02315000]  Winding3=[33.333, 0.00010000, 0.00010000]  Saturation=[ 0,0 ; 0.0024,1.2 ; 1.0,1.52 ]  CoreLoss=[500]  BreakLoop=on  DiscreteSolver=Trapezoidal iterative  DataType=off  InitialFlux=0.429801202991945  TransfoNumber=1
  VT C1 : powerlib/Elements/Saturable Transformer  ThreeWindings=on  Hysteresis=off  DataFile='hysteresis.mat'  Measurements=None  UNITS=pu  NominalPower=[600, 50]  Winding1=[5773.503, 0.00562500, 0.02315000]  Winding2=[57.735, 0.00562500, 0.02315000]  Winding3=[33.333, 0.00010000, 0.00010000]  Saturation=[ 0,0 ; 0.0024,1.2 ; 1.0,1.52 ]  CoreLoss=[500]  BreakLoop=on  DiscreteSolver=Trapezoidal iterative  DataType=off  InitialFlux=24.1850252874139  TransfoNumber=1
  A : PMIOPort  Side=Left
  B : PMIOPort  Port=2  Side=Left
  C : PMIOPort  Port=3  Side=Left
  Uabc1 : Outport
  Uabc2 : Outport  Port=2
  3U0 : Outport  Port=3
  wires:
  Mux3/1 -> Uabc2/1
  U0:1/1 -> 3U0/1
  Mux2/1 -> Uabc1/1
  U C:4/1 -> Mux3/3
  U B:4/1 -> Mux3/2
  U A:4/1 -> Mux3/1
  U C:3/1 -> Mux2/3
  U B:3/1 -> Mux2/2
  U A:3/1 -> Mux2/1
  connections:
  VT C1/RConn4 -- U0:1/LConn2 -- Ground4/LConn1
  U A:4/LConn2 -- U B:4/LConn2 -- U C:4/LConn2 -- R Load A1/RConn1 -- R Load B1/RConn1 -- R Load C1/RConn1 -- VT C1/RConn2 -- VT B1/RConn2 -- VT A1/RConn2
  VT B1/RConn1 -- R Load B1/LConn1 -- U B:4/LConn1
  VT C1/RConn1 -- R Load C1/LConn1 -- U C:4/LConn1
  VT B1/LConn1 -- U B:3/LConn1 -- B/RConn1
  VT C1/LConn1 -- U C:3/LConn1 -- C/RConn1
  VT A1/RConn1 -- R Load A1/LConn1 -- U A:4/LConn1
  U A:3/LConn1 -- VT A1/LConn1 -- A/RConn1
  Ground3/LConn1 -- U C:3/LConn2 -- VT B1/LConn2 -- U B:3/LConn2 -- VT A1/LConn2 -- U A:3/LConn2 -- VT C1/LConn2
  VT B1/RConn4 -- VT C1/RConn3
  VT A1/RConn3 -- U0:1/LConn1
  VT A1/RConn4 -- VT B1/RConn3
